simulink model "test"  (R2017a)
settings: Solver=VariableStepAuto  StartTime=0.0  StopTime=inf  RelTol=1e-3
libraries: untitledlibrary x3, realtime_pacer_lib x1
settings Model: Creator=ibrahim  LastModifiedBy=ibrahim
settings DebuggingCC: SFNoUnconditionalDefaultTransitionDiag=none

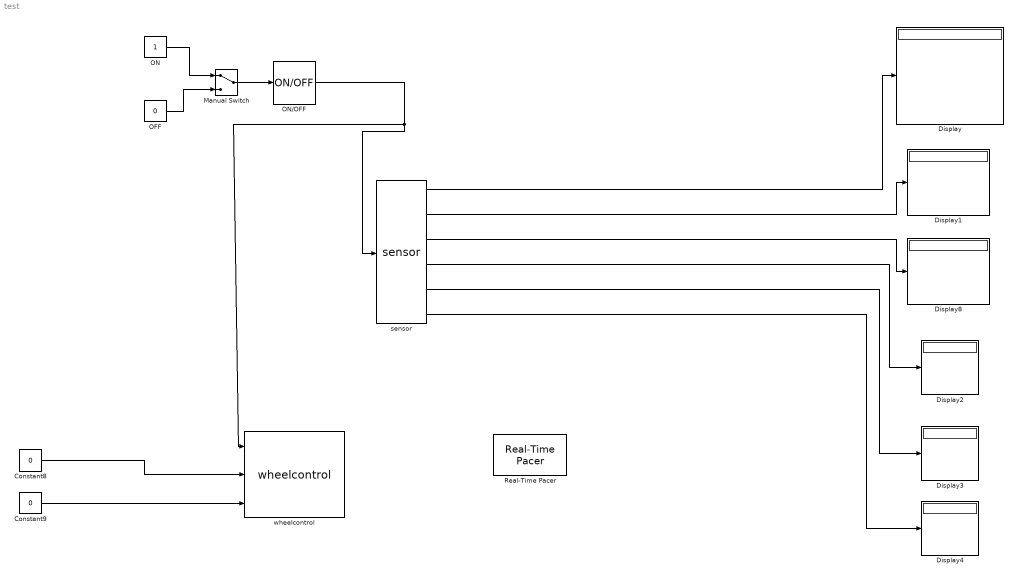
== system test ==
  Constant8 : Constant  Value=0
  Constant9 : Constant  Value=0
  Display{,1..4,8} (6 alike) : Display
  Manual Switch : ManualSwitch
  OFF : Constant  Value=0
  ON : Constant
  ON/OFF : untitledlibrary/ON//OFF
  Real-Time Pacer : realtime_pacer_lib/Real-Time Pacer  simTimePerRealTime=2
  sensor : untitledlibrary/sensor
  wheelcontrol : untitledlibrary/wheelcontrol  Priority=3
  wires:
  sensor/3 -> Display8/1
  Constant8/1 -> wheelcontrol/2
  Constant9/1 -> wheelcontrol/3
  sensor/2 -> Display1/1
  sensor/1 -> Display/1
  ON/OFF/1 -> sensor/1, wheelcontrol/1
  Manual Switch/1 -> ON/OFF/1
  ON/1 -> Manual Switch/1
  OFF/1 -> Manual Switch/2
  sensor/4 -> Display2/1
  sensor/5 -> Display3/1
  sensor/6 -> Display4/1
